simulink model "HDVSim_Hybrid_Truck_Platooning"  (R2018b)
settings: Solver=ode3  StartTime=0.0  StopTime=inf  FixedStep=sample_time  MaxStep=0.1  RelTol=1e-3  EnableMultiTasking=on
model workspace (MAT data in the model file):
  Anschaffungskosten = [3707764736; 2; 1; 1; 1; 1]
  Bat : struct (value not decoded)
  Driving_cycle = 18
  Eigenschaften = []
  Electric_Truck = 0
  Elektro_LKW = 0
  FuelCell : struct (value not decoded)
  Fueltype = 1
  Gewichte = [3707764736; 2; 1; 1; 2; 2]
  Hybrid_Truck = 0
  IZ12 = 3600
  Kraftstoff = 1
  M_el = 1000
  SOC_T_EM_completely_available = 0.5
  SOC_addition = 0.4
  SOC_el = 0.8
  SOC_target = 0.85
  Sailing_without_drag_torque = 0
  MCOS : class17 (value not decoded)
  TCO_Anhaenger = 1
  TCO_Trailer = 1
  T_distance_LPS_down = 250
  T_distance_LPS_up = 250
  VSim : struct (value not decoded)
  Vehicle = 'empty'
  WPT : struct (value not decoded)
  acquisition_costs = [3707764736; 2; 1; 1; 5; 5]
  addition_for_critical_slope = 0.01
  ambient : struct (value not decoded)
  auxiliary_consumers : struct (value not decoded)
  critical_altitude_difference = 50
  cycle : struct (value not decoded)
  dcycle = 18
  distance_1_PPC = 175
  distance_2_PPC = 200
  distance_PPC_altitude_difference = 10000
  driver : struct (value not decoded)
  em : struct (value not decoded)
  em_M_max = 1050
  engine : struct (value not decoded)
  final_drive : struct (value not decoded)
  ifElectric = 1
  ifOptimized = 0
  look_ahead_PPC = 250
  max_distance = 50000
  name = 'Verbrauchssimulation_Hybrid_LKW_Platooning'
  propertie = [3707764736; 2; 1; 1; 6; 6]
  prospective_cruise_control = 0
  sample_time = 0.1
  tank : struct (value not decoded)
  tires : struct (value not decoded)
  transmission : struct (value not decoded)
  v_PPC_delta = 2.77777777778
  v_max_electrical_drive_only = 13.8888888889
  vehicle : struct (value not decoded)
  vehicle_F_brake_max = 309890.14
  MCOS : class17 (value not decoded)
  x = 1
values from neighbouring files (symbols this model uses):
  transmission = Transmission_gearing(1, 1, false, false, final_drive.ratio)    [Parameterizing.m]
symbols that are objects in the model workspace (value not decoded): ambient, auxiliary_consumers, Bat, cycle, driver, em, engine, final_drive, tires, vehicle, WPT
undefined symbols (not defined in the file or in its folder): Ion, Lithium
libraries: simulink x23, powerlib x2, electricdrivelib x1
(part 3 of 3)

== stateflow chart HDVSim_Hybrid_Truck_Platooning/ECU/Chart ==
  state Hybrid_Truck
    state Accelerating
      state Boosting
        entry: BOOST = 1;
        during: u_ICE = 1; u_EM = (M_required - M_ICE_max) / M_EM_max; u_KB = 0; u_K = 0;
        exit: BOOST = 0;
      state load_point_lowering
        entry: LPlow = 1;
        during: u_ICE = (M_be_min - M_Drag) / (M_ICE_max - M_Drag); u_EM = (M_required - M_be_min) / M_EM_max; u_KB = 0; u_K = 0;
        exit: LPlow = 0;
      state ICE_driving
        during: u_ICE = (M_required - M_Drag) / (M_ICE_max - M_Drag); u_EM = 0; u_KB = 0; u_K = 0;
      state load_point_increasing
        entry: LPincrease = 1;
        during: u_ICE = (M_be_min - M_Drag) / (M_ICE_max - M_Drag); u_EM = - (M_be_min - M_required) / M_EM_max; u_KB = 0; u_K = 0;
        exit: LPincrease = 0;
      state Electric_driving
        entry: el_driving = 1;
        during: u_ICE = 0;  u_EM = M_required/M_EM_max; u_KB = 0; u_K = 1; % (M_Drag) / (M_ICE_max - M_Drag);
        exit: el_driving= 0;
      (junction 274) -> Boosting [order 3] : [M_required > M_be_min + M_EM_max &&...
          | SOC > 0]
      Boosting -> ICE_driving [order 3] : [SOC == 0]
      Boosting -> load_point_lowering [order 1] : [M_required < M_be_min + M_EM_max &&...
          | SOC > 0]
      load_point_lowering -> Boosting [order 1] : [M_required > M_be_min + M_EM_max &&...
          | SOC > 0]
      (junction 274) -> load_point_lowering [order 5] : [M_required > (M_be_min + T_distance_LPS_down) &&...
          | M_required <= M_be_min + M_EM_max &&...
          | SOC > 0]
      load_point_lowering -> ICE_driving [order 2] : [SOC == 0 ||...
          | M_required < M_be_min + T_distance_LPS_down]
      ICE_driving -> load_point_lowering [order 2] : [M_required > M_be_min + T_distance_LPS_down &&...
          | SOC > 0]
      (default) -> (junction 274)
      (junction 274) -> ICE_driving [order 2]
      (junction 274) -> Electric_driving [order 1] : [v_current<v_max_electrical_drive_only && SOC>0]
      (junction 274) -> load_point_increasing [order 4] : [M_required < (M_be_min - T_distance_LPS_up) &&...
          | M_required >= M_be_min - M_EM_max &&...
          | SOC < SOC_target+addition_for_SOC]
      ICE_driving -> Electric_driving [order 4] : [v_current<v_max_electrical_drive_only && SOC>0]
      Electric_driving -> ICE_driving : [v_current>=v_max_electrical_drive_only || SOC == 0]
      ICE_driving -> load_point_increasing [order 1] : [M_required < M_be_min - T_distance_LPS_up &&...
          | M_required > M_be_min - M_EM_max &&...
          | SOC < SOC_target+addition_for_SOC]
      load_point_increasing -> ICE_driving [order 1] : [M_required > M_be_min - T_distance_LPS_up ||...
          | M_required < M_be_min - M_EM_max  ||...
          | SOC >= SOC_target+addition_for_SOC]
    state Braking
      state Braking1
        % Conventional braking
        during: u_KB = Driver_B; u_ICE = 0; u_EM = 0; u_K = 0;
      state Braking2
        % Regenerative braking, additionally possibly conventional braking
        entry: REKUP = 1;
        exit: REKUP = 0;
        state Braking3
          % Regenerative and conventional braking
          during: u_EM = -1; u_KB = (F_brake_required - F_brake_el_max) / vehicle_F_brake_max; u_ICE = 0; u_K = 0;
        state Braking4
          % Regenerative braking
          during: u_EM = -(F_brake_required / F_brake_el_max); u_KB = 0;  u_K = 1; u_ICE=(M_Drag) / (M_ICE_max - M_Drag);
        (junction 205) -> Braking3 [order 1] : [F_brake_required > F_brake_el_max]
        Braking4 -> Braking3 : [F_brake_required > F_brake_el_max]
        Braking3 -> Braking4 : [F_brake_required <= F_brake_el_max]
        (default) -> (junction 205)
        (junction 205) -> Braking4 [order 2] : [F_brake_required <= F_brake_el_max]
      (junction 201) -> Braking1 [order 1] : [SOC == 1]
      Braking2 -> Braking1 : [SOC == 1]
      Braking1 -> Braking2 : [SOC < 1]
      (default) -> (junction 201)
      (junction 201) -> Braking2 [order 2]
    state Rolling
      entry: ROLL = 1;
      exit: ROLL = 0;
      state Rolling2
        during: u_ICE = (M_Drag) / (M_ICE_max - M_Drag); u_EM = 0; u_KB = 0; u_K = 1;
      state Rolling1
        during: u_EM = 0; u_ICE = 0; u_KB = 0; u_K = 0;
      (default) -> Rolling1
      Rolling1 -> Rolling2 : [Sailing_without_drag_torque == 1 && after(1,sec)]
    ICE_driving -> Rolling [order 3] : [Driver_M == 0 && Driver_B == 0]
    (default) -> (junction 206)
    (junction 206) -> Accelerating [order 1] : [Driver_M > 0 && Driver_B == 0]
    (junction 206) -> Braking [order 3] : [Driver_B > 0 && Driver_M == 0]
    (junction 206) -> Rolling [order 2]
    load_point_increasing -> Rolling [order 2] : [Driver_M == 0 && Driver_B == 0]
    Braking -> Accelerating [order 1] : [Driver_M > 0 && Driver_B == 0]
    Accelerating -> Braking : [Driver_B > 0 && Driver_M == 0]
    Rolling -> Accelerating [order 2] : [Driver_M > 0 && Driver_B == 0]
    Rolling -> Braking [order 1] : [Driver_B > 0 && Driver_M == 0]
    Braking -> Rolling [order 2] : [Driver_M == 0 && Driver_B == 0]
  state Conventional_Truck
    state Accelerating_conventional
      during: u_ICE = Driver_M; u_KB = 0; u_EM = 0; u_K = 0;
    state Braking_conventional
      during: u_ICE = 0; u_KB = Driver_B; u_EM = 0; u_K = 0;
    state Rolling_conventional
      during: u_ICE = 0; u_KB = 0; u_EM = 0; u_K = 0;
    Accelerating_conventional -> Rolling_conventional [order 2] : [Driver_M == 0 && Driver_B == 0]
    (junction 218) -> Accelerating_conventional [order 1] : [Driver_M > 0 && Driver_B == 0]
    Rolling_conventional -> Accelerating_conventional [order 2] : [Driver_M > 0 && Driver_B == 0]
    Braking_conventional -> Accelerating_conventional [order 1] : [Driver_M > 0 && Driver_B == 0]
    Accelerating_conventional -> Braking_conventional [order 1] : [Driver_B > 0 && Driver_M == 0]
    (default) -> (junction 218)
    (junction 218) -> Braking_conventional [order 2] : [Driver_B > 0 && Driver_M == 0]
    (junction 218) -> Rolling_conventional [order 3]
    Rolling_conventional -> Braking_conventional [order 1] : [Driver_B > 0 && Driver_M == 0]
    Braking_conventional -> Rolling_conventional [order 2] : [Driver_M == 0 && Driver_B == 0]
  Boosting -> Rolling [order 2] : [Driver_M == 0 && Driver_B == 0]
  load_point_lowering -> Rolling [order 3] : [Driver_M == 0 && Driver_B == 0]
  (junction 222) -> Hybrid_Truck [order 1] : [Hybrid_Truck == 1]
  (default) -> (junction 222)
  (junction 222) -> Conventional_Truck [order 2] : [Hybrid_Truck ~= 1]
  data: u_EM output; u_ICE output; Driver_M input; Driver_B input; SOC input; M_ICE_max input; M_EM_max input; M_required input; M_be_min input; M_Drag input; M_NV input; u_K output; F_brake_required input; F_brake_el_max input; u_KB output; SOC_target parameter; Hybrid_Truck parameter; BOOST output; LPlow output; LPincrease output; ROLL output; REKUP output; v_current input; el_driving output; v_max_electrical_drive_only parameter double; T_distance_LPS_down parameter double; T_distance_LPS_up parameter double; Sailing_without_drag_torque parameter double; addition_for_SOC input; vehicle_F_brake_max constant double =vehicle.F_brake_max; em_M_max constant double =em.M_max

== stateflow chart HDVSim_Hybrid_Truck_Platooning/Active cruise control/Chart ==
  state Incline
    entry: Signal_incline = 1;
    exit: Signal_incline = 0;
  state Even
  state Decline
    entry: Signal_decline = 1;
    exit: Signal_decline = 0;
  Even -> Incline [order 2] : [look_ahead_PPC > critical_incline &&...
      | look_ahead_PPC+distance_PPC > critical_incline &&...
      | prospective_cruise_control == 1]
  Incline -> Even : [incline_0 < critical_incline &&...
      | incline_100 < critical_incline &&...
      | incline_200 < critical_incline &&...
      | incline_300 < critical_incline &&...
      | incline_400 < critical_incline &&...
      | incline_500 < critical_incline &&...
      | Distance_covered > look_ahead_PPC+distance_PPC]
  (default) -> Even
  Even -> Decline [order 1] : [(Acceleration_0 +...
      | Acceleration_50 +...
      | Acceleration_100 +...
      | Acceleration_150 +...
      | Acceleration_200)/5 >= -(v_max_cycle/distance_2_PPC*v_PPC_delta) &&...
      | (Acceleration_250 +...
      | Acceleration_300 +...
      | Acceleration_350 +...
      | Acceleration_400 +...
      | Acceleration_450)/5 >= (v_max_cycle/distance_2_PPC*v_PPC_delta) &&...
      | Driver_M > 0 &&...
      | prospective_cruise_control == 1 &&...
      | v_current >= 60/3.6]
  Decline -> Even : [Distance_covered_2 > 450 ||...
      | Driver_B > 0]
  data: critical_incline input; Acceleration_0 input; Acceleration_50 input; Acceleration_100 input; Acceleration_150 input; Acceleration_200 input; Acceleration_250 input; Acceleration_300 input; Acceleration_350 input; Acceleration_400 input; Acceleration_450 input; incline_0 input; incline_100 input; incline_200 input; incline_300 input; incline_400 input; incline_500 input; incline_distance_look_ahead_min input; incline_distance_look_ahead_max input; Driver_M input; Driver_B input; Distance_covered input; Distance_covered_2 input; Signal_incline output double; Signal_decline output double; prospective_cruise_control constant double =preditiveCruiseControl; look_ahead constant double; v_PPC_delta constant double; v_max_cycle constant double; distance constant double; distance_2_PPC constant double; distance_PPC constant double; look_ahead_PPC constant double; v_current input

== stateflow chart HDVSim_Hybrid_Truck_Platooning/Transmission/Shifting strategy ==
  state gear_state [parallel]
    settings: executionOrder=1
    state gear016
      entry: gear=16;
    state gear015
      entry: gear=15;
    state gear014
      entry: gear=14;
    state gear013
      entry: gear=13;
    state gear012
      entry: gear=12;
    state gear011
      entry: gear=11;
    state gear010
      entry: gear=10;
    state gear09
      entry: gear=9;
    state gear08
      entry: gear=8;
    state gear07
      entry: gear=7;
    state gear06
      entry: gear=6;
    state gear05
      entry: gear=5;
    state gear04
      entry: gear=4;
    state gear03
      entry: gear=3;
    state gear02
      entry: gear=2;
    state gear01
      entry: gear=1;
    gear015 -> gear016 [order 3] : TWO_UP
    gear016 -> gear014 [order 2] : TWO_DOWN
    gear014 -> gear016 [order 3] : TWO_UP
    (junction 349) -> gear016 [order 16] : [init_gear==16]
    gear016 -> gear015 [order 1] : DOWN
    gear015 -> gear016 [order 1] : UP
    gear015 -> gear013 [order 4] : TWO_DOWN
    (junction 349) -> gear015 [order 15] : [init_gear==15]
    gear013 -> gear015 [order 3] : TWO_UP
    gear015 -> gear014 [order 2] : DOWN
    gear014 -> gear015 [order 1] : UP
    gear014 -> gear012 [order 4] : TWO_DOWN
    gear012 -> gear014 [order 4] : TWO_UP
    (junction 349) -> gear014 [order 14] : [init_gear==14]
    gear014 -> gear013 [order 2] : DOWN
    gear013 -> gear014 [order 1] : UP
    gear011 -> gear013 [order 4] : TWO_UP
    gear013 -> gear011 [order 4] : TWO_DOWN
    (junction 349) -> gear013 [order 13] : [init_gear==13]
    gear013 -> gear012 [order 2] : DOWN
    gear012 -> gear013 [order 3] : UP
    (junction 349) -> gear012 [order 12] : [init_gear==12]
    gear010 -> gear012 [order 4] : TWO_UP
    gear012 -> gear010 [order 2] : TWO_DOWN
    gear012 -> gear011 [order 1] : DOWN
    gear011 -> gear012 [order 1] : UP
    gear011 -> gear09 [order 3] : TWO_DOWN
    gear09 -> gear011 [order 4] : TWO_UP
    (junction 349) -> gear011 [order 11] : [init_gear==11]
    gear011 -> gear010 [order 2] : DOWN
    gear010 -> gear011 [order 1] : UP
    gear08 -> gear010 [order 4] : TWO_UP
    gear010 -> gear08 [order 3] : TWO_DOWN
    (junction 349) -> gear010 [order 10] : [init_gear==10]
    gear010 -> gear09 [order 2] : DOWN
    gear09 -> gear010 [order 1] : UP
    gear07 -> gear09 [order 4] : TWO_UP
    gear09 -> gear07 [order 3] : TWO_DOWN
    (junction 349) -> gear09 [order 9] : [init_gear==9]
    gear09 -> gear08 [order 2] : DOWN
    gear08 -> gear09 [order 2] : UP
    gear06 -> gear08 [order 4] : TWO_UP
    gear08 -> gear06 [order 3] : TWO_DOWN
    (junction 349) -> gear08 [order 8] : [init_gear==8]
    gear08 -> gear07 [order 1] : DOWN
    gear07 -> gear08 [order 3] : UP
    gear07 -> gear05 [order 2] : TWO_DOWN
    gear05 -> gear07 [order 4] : TWO_UP
    (junction 349) -> gear07 [order 7] : [init_gear==7]
    gear07 -> gear06 [order 1] : DOWN
    gear06 -> gear07 [order 3] : UP
    (junction 349) -> gear06 [order 6] : [init_gear==6]
    gear06 -> gear04 [order 2] : TWO_DOWN
    (junction 349) -> gear01 [order 1] : [init_gear==1]
    (junction 349) -> gear05 [order 5] : [init_gear==5]
    gear04 -> gear06 [order 3] : TWO_UP
    (junction 349) -> gear02 [order 2] : [init_gear==2]
    (junction 349) -> gear04 [order 4] : [init_gear==4]
    (junction 349) -> gear03 [order 3] : [init_gear==3]
    gear06 -> gear05 [order 1] : DOWN
    gear05 -> gear06 [order 1] : UP
    gear05 -> gear03 [order 3] : TWO_DOWN
    gear03 -> gear05 [order 3] : TWO_UP
    gear05 -> gear04 [order 2] : DOWN
    gear04 -> gear05 [order 1] : UP
    gear04 -> gear02 [order 4] : TWO_DOWN
    gear02 -> gear04 [order 3] : TWO_UP
    gear04 -> gear03 [order 2] : DOWN
    gear03 -> gear04 [order 1] : UP
    gear01 -> gear03 [order 2] : TWO_UP
    gear03 -> gear01 [order 4] : TWO_DOWN
    gear03 -> gear02 [order 2] : DOWN
    gear02 -> gear03 [order 1] : UP
    gear02 -> gear01 [order 4] : TWO_DOWN
    gear02 -> gear01 [order 2] : DOWN
    gear01 -> gear02 [order 1] : UP
  state selection_state [parallel]
    settings: executionOrder=2
    state upshift2
      entry: TWO_UP;
      exit: wait_state.WAIT;
    state upshift1
      entry: UP;
      exit: wait_state.WAIT;
    note: 2: UP due to recommendation
        | 3: UP due to speed max
    state steady_state
    note: 1: DOWN due to recommendation
        | 4: DOWN due to torque maximum
        | 5: DOWN due to speed min
    state downshift1
      entry: DOWN;
      exit: wait_state.WAIT;
    state downshift2
      entry: TWO_DOWN;
      exit: wait_state.WAIT;
    upshift2 -> steady_state
    (junction 405) -> upshift2 [order 1] : [recommend_down_2higher==0]
    (junction 405) -> upshift1 [order 2] : [recommend_down_2higher==1]
    (junction 404) -> (junction 405) [order 1] : [check_torque_reserve_2higher==1]
    (junction 404) -> upshift1 [order 2] : [check_torque_reserve_2higher==0]
    (junction 403) -> (junction 404) [order 1] : [check_n_min_2higher==1 && check_M_max_2higher==1]
    (junction 403) -> upshift1 [order 2] : [check_n_min_2higher==0 || check_M_max_2higher==0]
    (junction 380) -> (junction 403) [order 1] : [recommend_up_1higher==1 && gear<=z-2]
    (junction 380) -> upshift1 [order 2] : [recommend_up_1higher==0 || gear>z-2]
    steady_state -> upshift1 [order 3] : [check_n_max_now==0 && gear<=z-1]
    upshift1 -> steady_state
    steady_state -> (junction 380) [order 2] : [(recommend_up_now==1 && check_n_max_now==1) && check_n_min_1higher==1 && check_M_max_1higher==1 && gear<=z-1 && waiting3s==0]
    (default) -> steady_state
    downshift1 -> steady_state
    downshift2 -> steady_state
    steady_state -> (junction 367) [order 1] : [(recommend_down_now==1 && check_M_max_now==1 && check_n_min_now==1) && check_n_max_1lower==1 && gear>=2 && waiting3s==0]
    steady_state -> downshift1 [order 4] : [(check_M_max_now==0 && check_n_min_now==1) && check_n_max_1lower==1 &&gear>=2 && check_n_min_now==1 && waiting3s==0]
    steady_state -> downshift1 [order 5] : [(check_n_min_now==0)&& gear>3]
    (junction 367) -> downshift1 [order 1] : [recommend_down_1lower==0 || gear<3]
    (junction 367) -> (junction 394) [order 2] : [recommend_down_1lower==1 && gear>=3]
    (junction 394) -> downshift1 [order 2] : [check_n_max_2lower==0]
    (junction 394) -> (junction 397) [order 1] : [check_n_max_2lower==1]
    (junction 397) -> downshift1 [order 2] : [recommend_up_2lower==1]
    (junction 397) -> downshift2 [order 1] : [recommend_up_2lower==0]
  state wait_state [parallel]
    settings: executionOrder=3
    state shifting_ready
      entry: waiting3s=0;
    state wait3s
      entry: waiting3s=1;
    shifting_ready -> wait3s : WAIT
    (default) -> shifting_ready
    wait3s -> shifting_ready : after(3,sec)
  (default) -> (junction 349)
  data: gear output double; waiting3s local double; init_gear input double; z input double; recommend_down_2higher input boolean; recommend_down_1higher input boolean; recommend_down_now input boolean; recommend_down_1lower input boolean; recommend_down_2llower input boolean; recommend_up_2higher input boolean; recommend_up_1higher input boolean; recommend_up_now input boolean; recommend_up_1lower input boolean; recommend_up_2lower input boolean; check_n_min_2higher input boolean; check_n_min_1higher input boolean; check_n_min_now input boolean; check_n_min_1lower input boolean; check_n_min_2lower input boolean; check_n_max_2higher input boolean; check_n_max_1higher input boolean; check_n_max_now input boolean; check_n_max_1lower input boolean; check_n_max_2lower input boolean; check_M_max_2higher input boolean; check_M_max_1higher input boolean; check_M_max_now input boolean; check_M_max_1lower input boolean; check_M_max_2lower input boolean; check_torque_reserve_2higher input boolean; check_torque_reserve_2lower input boolean
  events: WAIT local EITHER_EDGE_EVENT; DOWN local EITHER_EDGE_EVENT; TWO_DOWN local EITHER_EDGE_EVENT; TWO_UP local EITHER_EDGE_EVENT; UP local EITHER_EDGE_EVENT

== matlab function HDVSim_Hybrid_Truck_Platooning/Transmission/Determine when shifting occurs/Gear change recommendation/recommend_down_calc_bsfc/MATLAB Function ==
  data: n input; g_1 output; M_max input; n_1 input; n_3 input
function g_1 = fcn(n,M_max,n_1,n_3)
%#codegen

g_1 = M_max / (n_3 - n_1) * (n - n_1);

== matlab function HDVSim_Hybrid_Truck_Platooning/Transmission/Determine when shifting occurs/Gear change recommendation/recommend_up_calc_bsfc/MATLAB Function1 ==
  data: n input; g_2 output; M_max input; n_6 input; n_2 input
function g_2 = fcn(n,M_max,n_6,n_2)
%#codegen

g_2 = M_max / (n_6 - n_2) * (n - n_2);

== stateflow chart HDVSim_Hybrid_Truck_Platooning/Active cruise control/Chart1 ==
  state Standard_SOC_target
  state SOC_target_increase
    entry: Signal_SOC_target_increase = 1;
    exit: Signal_SOC_target_increase = 0;
  (default) -> Standard_SOC_target
  Standard_SOC_target -> SOC_target_increase : [altitude_difference >= critical_altitude_difference]
  SOC_target_increase -> Standard_SOC_target : [Distance_covered >= distance_PPC_altitude_difference && increase_0 < 0]
  data: Signal_SOC_target_increase output; altitude_difference input; Distance_covered input; increase_0 input; distance_PPC_altitude_difference parameter; critical_altitude_difference parameter

== stateflow chart HDVSim_Hybrid_Truck_Platooning/ECU/Ausrollversuch/Chart1 ==
  state PassThrough_
    during: Out = In;
  state PassThrough_1
    during: Out = In;
  state Hold1
    during: Out = 0;
  (default) -> PassThrough_
  PassThrough_ -> PassThrough_1 : [v_current >= 80/3.6]
  PassThrough_1 -> Hold1 : after(10, sec)
  data: In input; Out output; v_current input

== stateflow chart HDVSim_Hybrid_Truck_Platooning/ECU/Ausrollversuch/Chart2 ==
  state PassThrough_
    during: Out = In;
  state PassThrough_1
    during: Out = In;
  state Hold1
    during: Out = 0;
  (default) -> PassThrough_
  PassThrough_ -> PassThrough_1 : [v_current >= 80/3.6]
  PassThrough_1 -> Hold1 : after(10, sec)
  data: In input; Out output; v_current input
